simulink model "model_real_int"  (R2015a)
settings: Solver=ode3  StartTime=0.0  StopTime=30  RelTol=1e-3
values from neighbouring files (symbols this model uses):
  K = dlqr(A, B, Q, R)    [teste_integrador.m]
  Ke = -3.922    [teste_integrador.m]
  Kp = 34.453    [teste_integrador.m]
  M = dlqe(A, G, C, Qw, Rw)    [teste_integrador.m]
  Nbar = Nu+K*Nx    [teste_integrador.m]
undefined symbols (not defined in the file or in its folder): A, B, C, MIO, National_Instruments, PCI, T
libraries: sldrtlib x2
settings Model: ExtModeTrigDuration=20000  Creator=alunos  LastModifiedBy=alunos
settings DataIOCC: LimitDataPoints=off
settings HardwareCC: ProdIntDivRoundTo=Zero  ProdEndianess=LittleEndian  ProdHWDeviceType=Intel->x86/Pentium  TargetIntDivRoundTo=Zero  TargetEndianess=LittleEndian  TargetHWDeviceType=Intel->x86/Pentium
settings RTWCC: SystemTargetFile=rtwin.tlc  TemplateMakefile=rtwin.tmf  Description=Simulink Desktop Real-Time  RTWCompilerOptimization=on
settings CodeAppCC: MaxIdLength=95
settings RTWinTargetCC: TargetPreCompLibLocation=C:\Program Files\MATLAB\R2015a\toolbox\sldrt\lib\win32

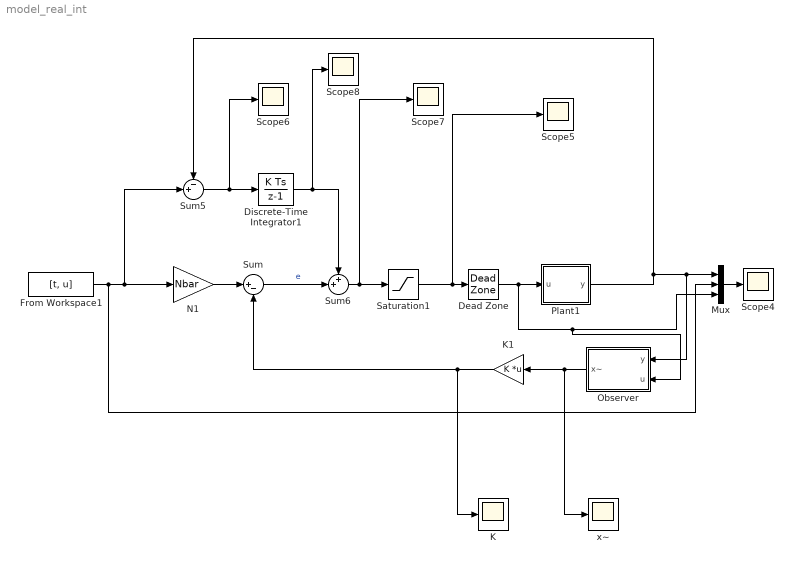
== system model_real_int ==
  Dead Zone : DeadZone  LowerValue=-0.28  UpperValue=0.3  SaturateOnIntegerOverflow=on
  Discrete-Time Integrator1 : DiscreteIntegrator  gainval=Ki  InitialConditionSetting=State (most efficient)  SampleTime=-1
  From Workspace1 : FromWorkspace  VariableName=[t, u]  SampleTime=T
  K : Scope
      settings: SaveName=test_controller
  K1 : Gain  Gain=K  Multiplication=Matrix(K*u)
  Mux : Mux  Inputs=3
  N1 : Gain  Gain=Nbar
  Observer : Subsystem
  Plant1 : Subsystem
  Saturation1 : Saturate  UpperLimit=10  LowerLimit=-10
  Scope{4..8} (5 alike) : Scope
      Scope4 settings: YMin=-15  YMax=15  SaveName=test_controller5
      Scope5 settings: SaveName=test_controller6
      Scope6 settings: SaveName=test_controller7
      Scope7 settings: SaveName=test_controller8
      Scope8 settings: SaveName=test_controller4
  Sum : Sum  Inputs=|+-
  Sum5 : Sum  Inputs=-+|
  Sum6 : Sum  Inputs=++|
  "x~ " : Scope
      settings: SaveName=test_controller1
  wires:
  K1/1 -> K/1, Sum/2
  Plant1/1(y) -> Sum5/1, Observer/1(y), Mux/1
  Mux/1 -> Scope4/1
  Saturation1/1 -> Dead Zone/1, Scope5/1
  Sum5/1 -> Discrete-Time Integrator1/1, Scope6/1
  From Workspace1/1 -> Sum5/2, N1/1, Mux/2
  N1/1 -> Sum/1
  Observer/1(x~) -> "x~ "/1, K1/1
  Sum6/1 -> Scope7/1, Saturation1/1
  Sum/1 -> Sum6/2  "e"
  Discrete-Time Integrator1/1 -> Scope8/1, Sum6/1
  Dead Zone/1 -> Plant1/1(u), Observer/2(u), Mux/3

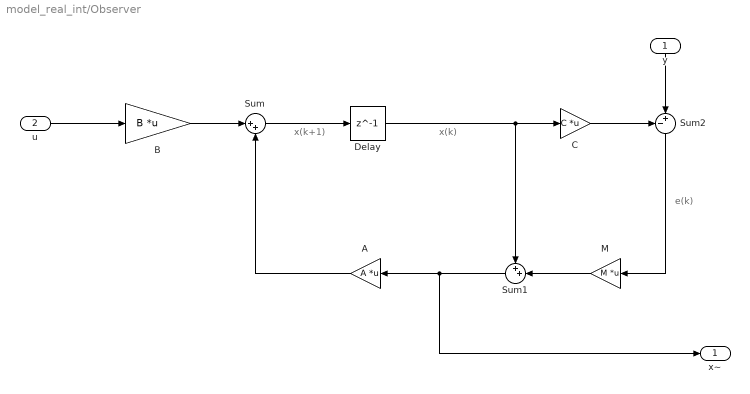
== system model_real_int/Observer ==
  note: e(k)
  note: x(k)
  note: x(k+1)
  y : Inport  PortDimensions=1
  u : Inport  Port=2
  A : Gain  Gain=A  Multiplication=Matrix(K*u)
  B : Gain  Gain=B  Multiplication=Matrix(K*u) (u vector)
  C : Gain  Gain=C  Multiplication=Matrix(K*u)
  Delay : Delay  DelayLength=1  InitialCondition=[0;0;0;0]
  M : Gain  Gain=M  Multiplication=Matrix(K*u) (u vector)
  Sum : Sum  Inputs=|++
  Sum1 : Sum  Inputs=++|
  Sum2 : Sum  Inputs=-+|
  x~ : Outport  PortDimensions=[4,1]
  wires:
  Sum/1 -> Delay/1
  C/1 -> Sum2/1
  Sum2/1 -> M/1
  Delay/1 -> C/1, Sum1/1
  M/1 -> Sum1/2
  A/1 -> Sum/2
  y/1 -> Sum2/2
  u/1 -> B/1
  Sum1/1 -> x~/1, A/1
  B/1 -> Sum/1

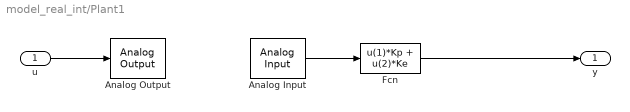
== system model_real_int/Plant1 ==
  u : Inport
  Analog Input : sldrtlib/Analog Input  SampleTime=T  MaxMissedTicks=10  ShowMissedTicks=off  YieldWhenWaiting=off  DrvName=National_Instruments/PCI-MIO-16E-4  DrvAddress=4294967295  DrvOptions=[0 0 0 0 0 0]  Channels=1:3  RangeMode=1  VoltRange=1  DataType=1
      settings: AttributesFormatString=National Instruments\nPCI-MIO-16E-4 [auto]
  Analog Output : sldrtlib/Analog Output  SampleTime=T  MaxMissedTicks=10  ShowMissedTicks=off  YieldWhenWaiting=off  DrvName=National_Instruments/PCI-MIO-16E-4  DrvAddress=4294967295  DrvOptions=[0 0 0 0 0 0]  Channels=1  RangeMode=1  VoltRange=1  InitialValue=0  FinalValue=0
      settings: AttributesFormatString=National Instruments\nPCI-MIO-16E-4 [auto]
  Fcn : Fcn  Expr=u(1)*Kp + u(2)*Ke
  y : Outport
  wires:
  Analog Input/1 -> Fcn/1
  u/1 -> Analog Output/1
  Fcn/1 -> y/1
